simulink model "PID_base_simulink"  (R2022b)
settings: Solver=VariableStepAuto  StartTime=0.0  StopTime=10.0  RelTol=1e-3
undefined symbols (not defined in the file): A1, A2, Be, f, k, kc1, kc2, kq1, kq2, M, V1, V2
libraries: simulink x1
settings Model: Creator=dsilva  LastModifiedBy=dsilva
settings DataIOCC: ReturnWorkspaceOutputs=off

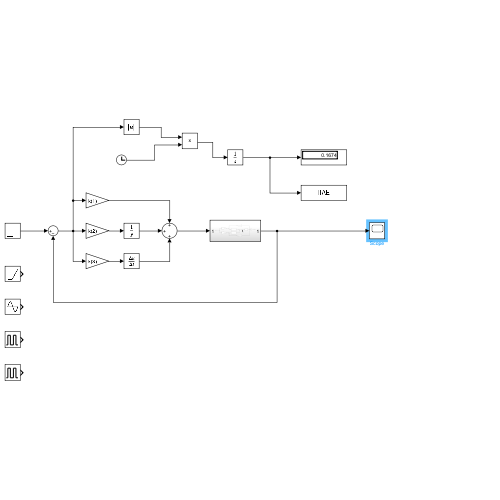
[thumbnail: Simulink's stored preview of the top-level diagram]
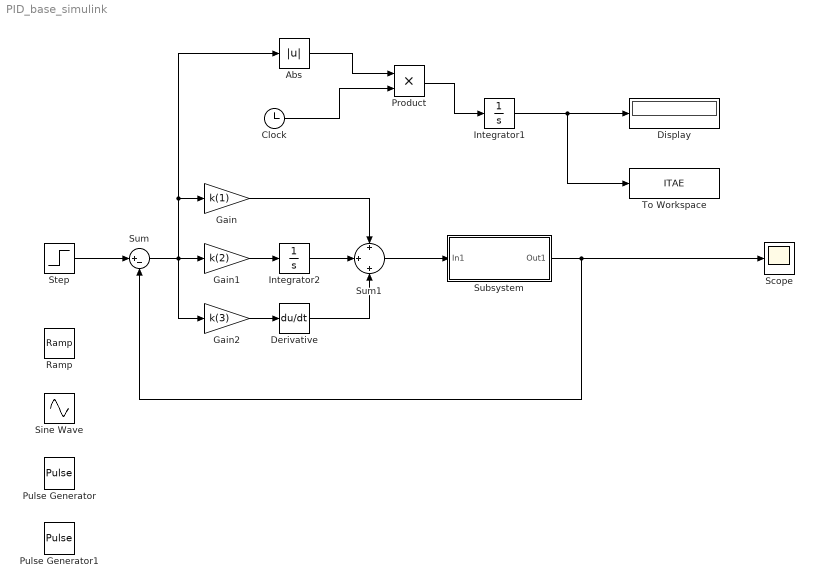
== system PID_base_simulink ==
  Abs : Abs  SaturateOnIntegerOverflow=off
  Clock : Clock
  Derivative : Derivative
  Display : Display
  Gain : Gain  Gain=k(1)
  Gain1 : Gain  Gain=k(2)
  Gain2 : Gain  Gain=k(3)
  Integrator1 : Integrator
  Integrator2 : Integrator
  Product : Product
  Pulse Generator : DiscretePulseGenerator  PulseType=Time based  Period=10  PulseWidth=5
  Pulse Generator1 : DiscretePulseGenerator  PulseType=Time based  Period=10  PulseWidth=20
  Ramp : simulink/Sources/Ramp  slope=1  start=0  InitialOutput=0
  Scope : Scope
  Sine Wave : Sin  Frequency=2  SampleTime=0
  Step : Step  SampleTime=0
  Subsystem : Subsystem
  Sum : Sum  Inputs=|+-
  Sum1 : Sum  Inputs=+|+|+
  To Workspace : ToWorkspace  VariableName=ITAE  SampleTime=-1
  wires:
  Gain1/1 -> Integrator2/1
  Sum/1 -> Abs/1, Gain/1, Gain2/1, Gain1/1
  Gain2/1 -> Derivative/1
  Integrator1/1 -> To Workspace/1, Display/1
  Gain/1 -> Sum1/1
  Subsystem/1(Out1) -> Scope/1, Sum/2
  Integrator2/1 -> Sum1/2
  Abs/1 -> Product/1
  Derivative/1 -> Sum1/3
  Sum1/1 -> Subsystem/1(In1)
  Step/1 -> Sum/1
  Clock/1 -> Product/2
  Product/1 -> Integrator1/1

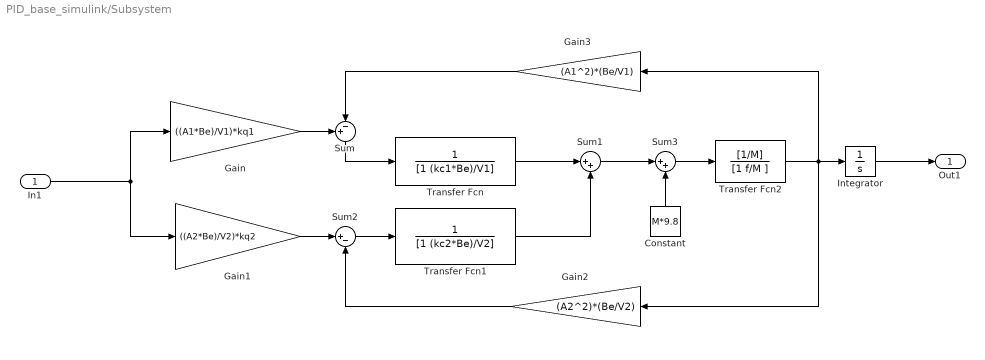
== system PID_base_simulink/Subsystem ==
  In1 : Inport
  Constant : Constant  Value=M*9.8
  Gain : Gain  Gain=((A1*Be)/V1)*kq1
  Gain1 : Gain  Gain=((A2*Be)/V2)*kq2
  Gain2 : Gain  Gain=(A2^2)*(Be/V2)
  Gain3 : Gain  Gain=(A1^2)*(Be/V1)
  Integrator : Integrator
  Sum : Sum  Inputs=+-|
  Sum1 : Sum  Inputs=|++
  Sum2 : Sum  Inputs=|+-
  Sum3 : Sum  Inputs=|++
  Transfer Fcn : TransferFcn  Denominator=[1 (kc1*Be)/V1]
  Transfer Fcn1 : TransferFcn  Denominator=[1 (kc2*Be)/V2]
  Transfer Fcn2 : TransferFcn  Numerator=[1/M]  Denominator=[1 f/M ]
  Out1 : Outport
  wires:
  Sum1/1 -> Sum3/1
  Constant/1 -> Sum3/2
  Gain1/1 -> Sum2/1
  Sum3/1 -> Transfer Fcn2/1
  Transfer Fcn2/1 -> Gain2/1, Gain3/1, Integrator/1
  Gain2/1 -> Sum2/2
  Sum2/1 -> Transfer Fcn1/1
  Transfer Fcn1/1 -> Sum1/2
  Transfer Fcn/1 -> Sum1/1
  In1/1 -> Gain/1, Gain1/1
  Integrator/1 -> Out1/1
  Sum/1 -> Transfer Fcn/1
  Gain3/1 -> Sum/2
  Gain/1 -> Sum/1
